simulink model "SETL2_TestLevel_2_MODEL_Training"  (R2017b)
settings: Solver=VariableStepAuto  StartTime=0.0  StopTime=25000000  MaxStep=200  RelTol=1e-3
model workspace (MAT data in the model file):
  Ba = 98.3523688074
  Br = 64.1345426034
  Bw = 39.6355439353
libraries: instrumentlib x2, svdutilitieslib x1
settings Model: Creator=Bruger  LastModifiedBy=koch

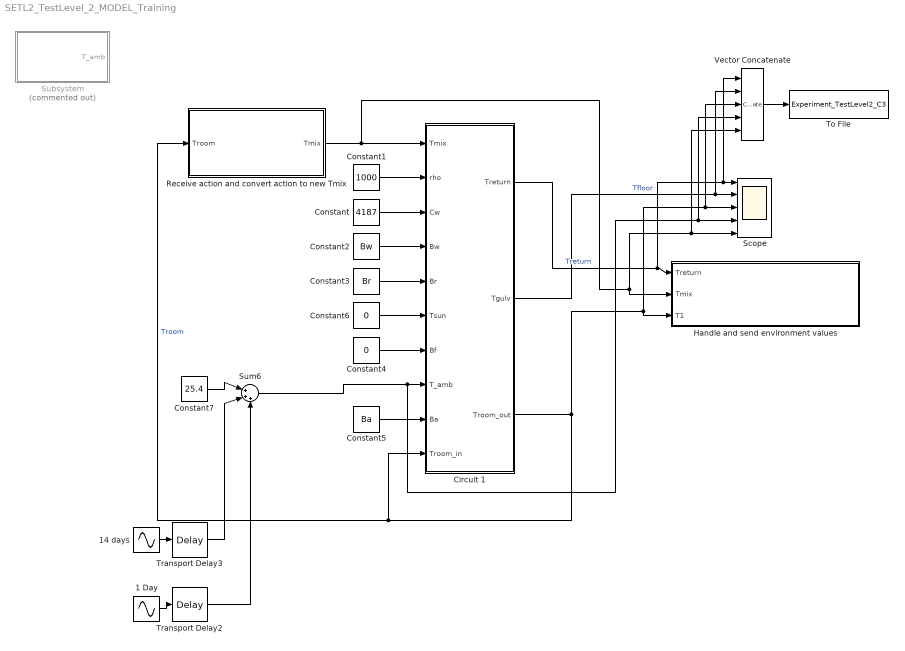
== system SETL2_TestLevel_2_MODEL_Training ==
  1 Day : Sin  Frequency=0.00014  SampleTime=0
  14 days : Sin  Frequency=0.00007272205216643  SampleTime=0
  Circuit 1 : Subsystem
  Constant : Constant  Value=4187
  Constant1 : Constant  Value=1000
  Constant2 : Constant  Value=Bw
  Constant3 : Constant  Value=Br
  Constant4 : Constant  Value=0
  Constant5 : Constant  Value=Ba
  Constant6 : Constant  Value=0
  Constant7 : Constant  Value=25.4
  Handle and send environment values : Subsystem
  Receive action and convert action to new Tmix : Subsystem
  Scope : Scope  NumInputPorts=5
  Subsystem : Subsystem  Commented=on
  Sum6 : Sum  Inputs=|+++
  To File : ToFile  Filename=Experiment_TestLevel2_C3  SaveFormat=Timeseries
  Transport Delay2 : TransportDelay  DelayTime=4000000
  Transport Delay3 : TransportDelay  DelayTime=3000000
  Vector Concatenate : Concatenate  NumInputs=5
  wires:
  Circuit 1/1(Treturn) -> Vector Concatenate/1, Scope/1, Handle and send environment values/1(Treturn)  "Treturn"
  Circuit 1/3(Troom_out) -> Vector Concatenate/3, Scope/3, Handle and send environment values/3(T1), Receive action and convert action to new Tmix/1(Troom), Circuit 1/10(Troom_in)  "Troom"
  Constant1/1 -> Circuit 1/2(rho)
  Constant/1 -> Circuit 1/3(Cw)
  Constant2/1 -> Circuit 1/4(Bw)
  Constant3/1 -> Circuit 1/5(Br)
  Constant6/1 -> Circuit 1/6(Tsun)
  Constant4/1 -> Circuit 1/7(Bf)
  Constant5/1 -> Circuit 1/9(Ba)
  Receive action and convert action to new Tmix/1(Tmix) -> Vector Concatenate/5, Scope/5, Handle and send environment values/2(Tmix), Circuit 1/1(Tmix)
  Vector Concatenate/1 -> To File/1
  Circuit 1/2(Tgulv) -> Vector Concatenate/2, Scope/2  "Tfloor"
  Transport Delay3/1 -> Sum6/2
  Constant7/1 -> Sum6/1
  14 days/1 -> Transport Delay3/1
  1 Day/1 -> Transport Delay2/1
  Transport Delay2/1 -> Sum6/3
  Sum6/1 -> Vector Concatenate/4, Scope/4, Circuit 1/8(T_amb)

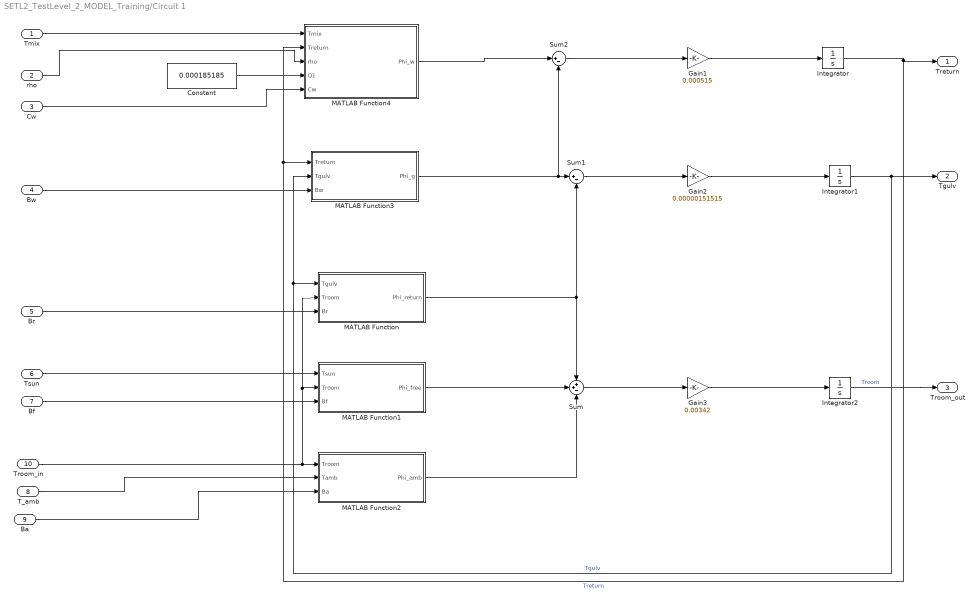
== system SETL2_TestLevel_2_MODEL_Training/Circuit 1 ==
  Tmix : Inport
  rho : Inport  Port=2
  Cw : Inport  Port=3
  Bw : Inport  Port=4
  Br : Inport  Port=5
  Tsun : Inport  Port=6
  Bf : Inport  Port=7
  T_amb : Inport  Port=8
  Ba : Inport  Port=9
  Troom_in : Inport  Port=10
  Constant : Constant  Value=0.000185185
  Gain1 : Gain  Gain=0.000515
  Gain2 : Gain  Gain=0.00000151515
  Gain3 : Gain  Gain=0.00342
  Integrator : Integrator  InitialCondition=25.5
  Integrator1 : Integrator  InitialCondition=25.5
  Integrator2 : Integrator  InitialCondition=25.5
  MATLAB Function : MATLAB Function  TreatAsAtomicUnit=on
  MATLAB Function1 : MATLAB Function  TreatAsAtomicUnit=on
  MATLAB Function2 : MATLAB Function  TreatAsAtomicUnit=on
  MATLAB Function3 : MATLAB Function  TreatAsAtomicUnit=on
  MATLAB Function4 : MATLAB Function  TreatAsAtomicUnit=on
  Sum : Sum  Inputs=++-
  Sum1 : Sum  Inputs=|+-
  Sum2 : Sum  Inputs=|+-
  Treturn : Outport
  Tgulv : Outport  Port=2
  Troom_out : Outport  Port=3
  wires:
  MATLAB Function1/1(Phi_free) -> Sum/2
  MATLAB Function4/1(Phi_w) -> Sum2/1
  Constant/1 -> MATLAB Function4/4(Q1)
  MATLAB Function2/1(Phi_amb) -> Sum/3
  Sum2/1 -> Gain1/1
  Bf/1 -> MATLAB Function1/3(Bf)
  Integrator1/1 -> MATLAB Function/1(Tgulv), MATLAB Function3/2(Tgulv), Tgulv/1  "Tgulv"
  Integrator2/1 -> Troom_out/1  "Troom"
  MATLAB Function3/1(Phi_g) -> Sum2/2, Sum1/1
  MATLAB Function/1(Phi_return) -> Sum/1, Sum1/2
  Bw/1 -> MATLAB Function3/3(Bw)
  Cw/1 -> MATLAB Function4/5(Cw)
  rho/1 -> MATLAB Function4/3(rho)
  Sum1/1 -> Gain2/1
  Gain1/1 -> Integrator/1
  Gain2/1 -> Integrator1/1
  Integrator/1 -> MATLAB Function4/2(Treturn), MATLAB Function3/1(Treturn), Treturn/1  "Treturn"
  Tsun/1 -> MATLAB Function1/1(Tsun)
  Gain3/1 -> Integrator2/1
  Ba/1 -> MATLAB Function2/3(Ba)
  Br/1 -> MATLAB Function/3(Br)
  Sum/1 -> Gain3/1
  Troom_in/1 -> MATLAB Function2/1(Troom), MATLAB Function/2(Troom), MATLAB Function1/2(Troom)
  Tmix/1 -> MATLAB Function4/1(Tmix)
  T_amb/1 -> MATLAB Function2/2(Tamb)

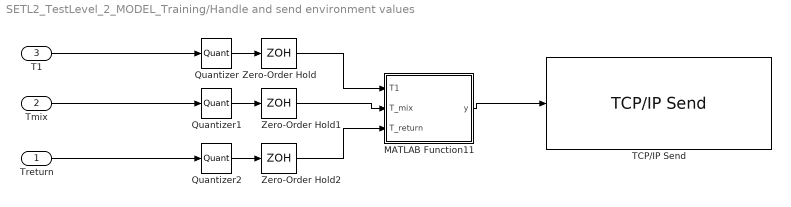
== system SETL2_TestLevel_2_MODEL_Training/Handle and send environment values ==
  Treturn : Inport
  Tmix : Inport  Port=2
  T1 : Inport  Port=3
  MATLAB Function11 : MATLAB Function  TreatAsAtomicUnit=on
  Quantizer : Quantizer  QuantizationInterval=0.01
  Quantizer1 : Quantizer  QuantizationInterval=0.01
  Quantizer2 : Quantizer  QuantizationInterval=0.01
  TCP/IP Send : instrumentlib/TCP//IP Send  Priority=2  Host=localhost  Port=50001  EnableBlockingMode=on  Timeout=10  ByteOrder=LittleEndian
      settings: SourceProductName=Instrument Control Toolbox
  Zero-Order Hold : ZeroOrderHold  SampleTime=-1
  Zero-Order Hold1 : ZeroOrderHold  SampleTime=-1
  Zero-Order Hold2 : ZeroOrderHold  SampleTime=-1
  wires:
  Quantizer1/1 -> Zero-Order Hold1/1
  Quantizer/1 -> Zero-Order Hold/1
  Quantizer2/1 -> Zero-Order Hold2/1
  Zero-Order Hold1/1 -> MATLAB Function11/2(T_mix)
  Zero-Order Hold/1 -> MATLAB Function11/1(T1)
  Zero-Order Hold2/1 -> MATLAB Function11/3(T_return)
  MATLAB Function11/1(y) -> TCP/IP Send/1
  Tmix/1 -> Quantizer1/1
  T1/1 -> Quantizer/1
  Treturn/1 -> Quantizer2/1

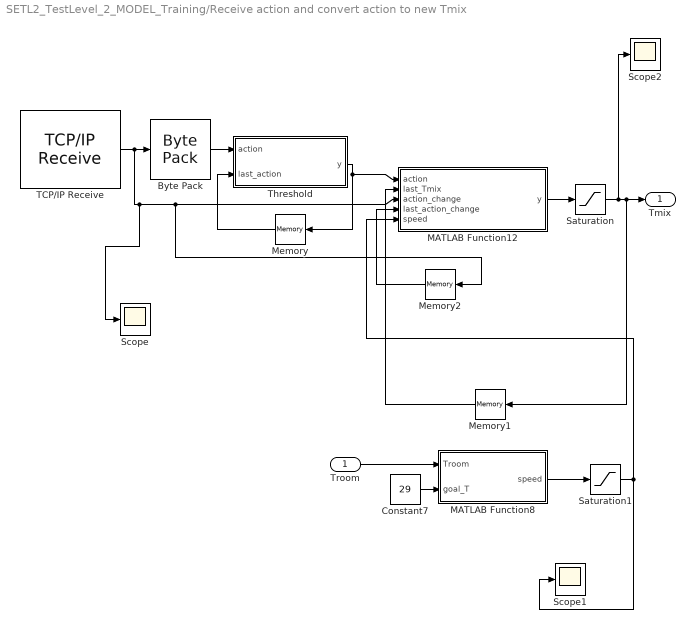
== system SETL2_TestLevel_2_MODEL_Training/Receive action and convert action to new Tmix ==
  Troom : Inport
  Byte Pack : svdutilitieslib/Byte Pack  datatypes={'uint8'}  byteAlign=1  blockPlatform=arduinoert
      settings: SourceProductName=Simulink Support Package for Arduino Hardware  SourceProductBaseCode=ARDUINO
  Constant7 : Constant  Value=29
  MATLAB Function12 : MATLAB Function  TreatAsAtomicUnit=on
  MATLAB Function8 : MATLAB Function  TreatAsAtomicUnit=on
  Memory : Memory
  Memory1 : Memory  InitialCondition=24
  Memory2 : Memory
  Saturation : Saturate  UpperLimit=60  LowerLimit=24
  Saturation1 : Saturate  UpperLimit=0.8  LowerLimit=0.005
  Scope : Scope
  Scope1 : Scope
  Scope2 : Scope
  TCP/IP Receive : instrumentlib/TCP//IP Receive  Host=localhost  Port=50000  DataSize=[1 1]  EnableBlockingMode=on  Timeout=15  SampleTime=50  DataType=uint8  ByteOrder=BigEndian
      settings: SourceProductName=Instrument Control Toolbox
  Threshold : MATLAB Function  TreatAsAtomicUnit=on
  Tmix : Outport
  wires:
  MATLAB Function12/1(y) -> Saturation/1
  TCP/IP Receive/1 -> Scope/1, Memory2/1, MATLAB Function12/3(action_change), Byte Pack/1
  Threshold/1(y) -> MATLAB Function12/1(action), Memory/1
  MATLAB Function8/1(speed) -> Saturation1/1
  Saturation1/1 -> Scope1/1, MATLAB Function12/5(speed)
  Memory/1 -> Threshold/2(last_action)
  Saturation/1 -> Scope2/1, Tmix/1, Memory1/1
  Byte Pack/1 -> Threshold/1(action)
  Constant7/1 -> MATLAB Function8/2(goal_T)
  Memory1/1 -> MATLAB Function12/2(last_Tmix)
  Troom/1 -> MATLAB Function8/1(Troom)
  Memory2/1 -> MATLAB Function12/4(last_action_change)

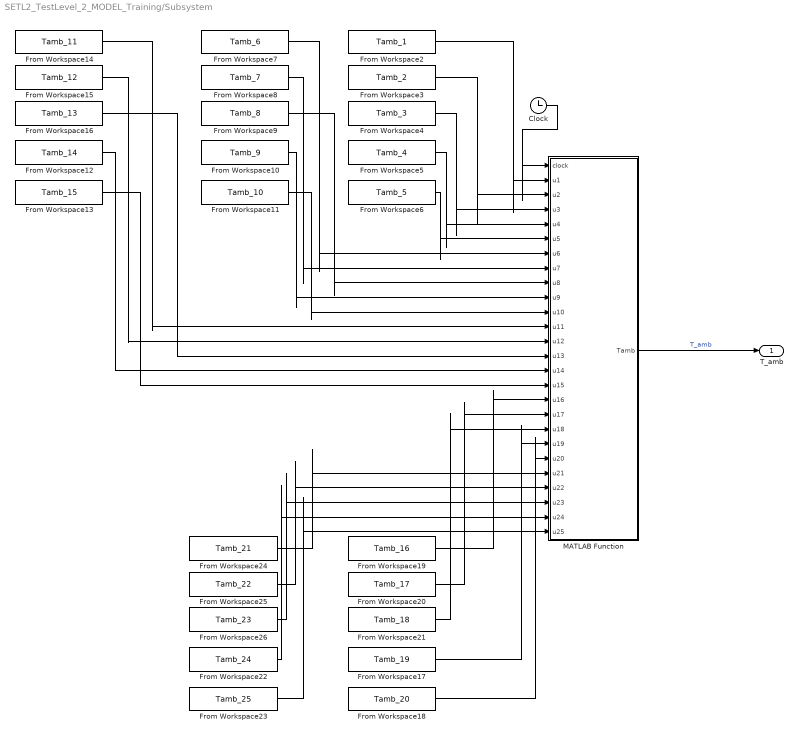
== system SETL2_TestLevel_2_MODEL_Training/Subsystem ==
  Clock : Clock
  From Workspace10 : FromWorkspace  VariableName=Tamb_9  SampleTime=0
  From Workspace11 : FromWorkspace  VariableName=Tamb_10  SampleTime=0
  From Workspace12 : FromWorkspace  VariableName=Tamb_14  SampleTime=0
  From Workspace13 : FromWorkspace  VariableName=Tamb_15  SampleTime=0
  From Workspace14 : FromWorkspace  VariableName=Tamb_11  SampleTime=0
  From Workspace15 : FromWorkspace  VariableName=Tamb_12  SampleTime=0
  From Workspace16 : FromWorkspace  VariableName=Tamb_13  SampleTime=0
  From Workspace17 : FromWorkspace  VariableName=Tamb_19  SampleTime=0
  From Workspace18 : FromWorkspace  VariableName=Tamb_20  SampleTime=0
  From Workspace19 : FromWorkspace  VariableName=Tamb_16  SampleTime=0
  From Workspace2 : FromWorkspace  VariableName=Tamb_1  SampleTime=0
  From Workspace20 : FromWorkspace  VariableName=Tamb_17  SampleTime=0
  From Workspace21 : FromWorkspace  VariableName=Tamb_18  SampleTime=0
  From Workspace22 : FromWorkspace  VariableName=Tamb_24  SampleTime=0
  From Workspace23 : FromWorkspace  VariableName=Tamb_25  SampleTime=0
  From Workspace24 : FromWorkspace  VariableName=Tamb_21  SampleTime=0
  From Workspace25 : FromWorkspace  VariableName=Tamb_22  SampleTime=0
  From Workspace26 : FromWorkspace  VariableName=Tamb_23  SampleTime=0
  From Workspace3 : FromWorkspace  VariableName=Tamb_2  SampleTime=0
  From Workspace4 : FromWorkspace  VariableName=Tamb_3  SampleTime=0
  From Workspace5 : FromWorkspace  VariableName=Tamb_4  SampleTime=0
  From Workspace6 : FromWorkspace  VariableName=Tamb_5  SampleTime=0
  From Workspace7 : FromWorkspace  VariableName=Tamb_6  SampleTime=0
  From Workspace8 : FromWorkspace  VariableName=Tamb_7  SampleTime=0
  From Workspace9 : FromWorkspace  VariableName=Tamb_8  SampleTime=0
  MATLAB Function : MATLAB Function  TreatAsAtomicUnit=on
  T_amb : Outport
  wires:
  Clock/1 -> MATLAB Function/1(clock)
  From Workspace3/1 -> MATLAB Function/3(u2)
  MATLAB Function/1(Tamb) -> T_amb/1  "T_amb"
  From Workspace22/1 -> MATLAB Function/25(u24)
  From Workspace6/1 -> MATLAB Function/6(u5)
  From Workspace4/1 -> MATLAB Function/4(u3)
  From Workspace7/1 -> MATLAB Function/7(u6)
  From Workspace18/1 -> MATLAB Function/21(u20)
  From Workspace16/1 -> MATLAB Function/14(u13)
  From Workspace15/1 -> MATLAB Function/13(u12)
  From Workspace5/1 -> MATLAB Function/5(u4)
  From Workspace9/1 -> MATLAB Function/9(u8)
  From Workspace13/1 -> MATLAB Function/16(u15)
  From Workspace11/1 -> MATLAB Function/11(u10)
  From Workspace14/1 -> MATLAB Function/12(u11)
  From Workspace20/1 -> MATLAB Function/18(u17)
  From Workspace12/1 -> MATLAB Function/15(u14)
  From Workspace10/1 -> MATLAB Function/10(u9)
  From Workspace25/1 -> MATLAB Function/23(u22)
  From Workspace24/1 -> MATLAB Function/22(u21)
  From Workspace26/1 -> MATLAB Function/24(u23)
  From Workspace8/1 -> MATLAB Function/8(u7)
  From Workspace19/1 -> MATLAB Function/17(u16)
  From Workspace23/1 -> MATLAB Function/26(u25)
  From Workspace21/1 -> MATLAB Function/19(u18)
  From Workspace17/1 -> MATLAB Function/20(u19)
  From Workspace2/1 -> MATLAB Function/2(u1)

== matlab function SETL2_TestLevel_2_MODEL_Training/Circuit 1/MATLAB Function1 ==
  data: Tsun input; Phi_free output; Troom input; Bf input
function Phi_free = fcn(Tsun,Troom,Bf)

Phi_free = Bf * ( Tsun-Troom)

== matlab function SETL2_TestLevel_2_MODEL_Training/Circuit 1/MATLAB Function ==
  data: Tgulv input; Phi_return output; Troom input; Br input
function Phi_return = fcn(Tgulv,Troom,Br)

Phi_return = Br * ( Tgulv-Troom)

== matlab function SETL2_TestLevel_2_MODEL_Training/Circuit 1/MATLAB Function2 ==
  data: Troom input; Tamb input; Phi_amb output; Ba input
function Phi_amb = fcn(Troom,Tamb,Ba)

Phi_amb = Ba * ( Troom-Tamb)

== matlab function SETL2_TestLevel_2_MODEL_Training/Circuit 1/MATLAB Function3 ==
  data: Treturn input; Tgulv input; Phi_g output; Bw input
function Phi_g= fcn(Treturn,Tgulv,Bw)

Phi_g = Bw * ( Treturn-Tgulv)

== matlab function SETL2_TestLevel_2_MODEL_Training/Circuit 1/MATLAB Function4 ==
  data: Tmix input; Treturn input; Phi_w output; rho input; Q1 input; Cw input
function Phi_w= fcn(Tmix,Treturn,rho,Q1,Cw)

Phi_w = rho*Q1 *Cw* ( Tmix-Treturn)

== matlab function SETL2_TestLevel_2_MODEL_Training/Subsystem/MATLAB Function ==
  data: clock input; Tamb output; u1 input; u2 input; u3 input; u4 input; u5 input; u6 input; u7 input; u8 input; u9 input; u10 input; u11 input; u12 input; u13 input; u14 input; u15 input; u16 input; u17 input; u18 input; u19 input; u20 input; u21 input; u22 input; u23 input; u24 input; u25 input
function Tamb = fcn(clock, u1, u2, u3, u4, u5, u6, u7, u8, u9, u10, u11, u12, u13, u14, u15, u16, u17, u18, u19, u20, u21, u22, u23, u24, u25)

if clock <= 1604445
    Tamb = 25.4375;
elseif 1604445 < clock <= 1604445*2
    Tamb = u2;
elseif 1604445*2 < clock <= 1604445*3
    Tamb = u3;
elseif 1604445*3 < clock <= 1604445*4
    Tamb = u4;
elseif 1604445*4 < clock <= 1604445*5
    Tamb = u5;
elseif 1604445*5 < clock <= 1604445*6
    Tamb = u6;
elseif 1604445*6 < clock <= 1604445*7
    Tamb = u7;
elseif 1604445*7 < clock <= 1604445*8
    Tamb = u8;
elseif 1604445*8 < clock <= 1604445*9
    Tamb = u9;
elseif 1604445*9 < clock <= 1604445*10
    Tamb = u10;
elseif 1604445*10 < clock <= 1604445*11
    Tamb = u11;
elseif 1604445*11 < clock <= 1604445*12
    Tamb = u12;
elseif 1604445*12 < clock <= 1604445*13
    Tamb = u13;
elseif 1604445*13 < clock <= 1604445*14
    Tamb = u14;
elseif 1604445*14 < clock <= 1604445*15
    Tamb = u15;
elseif 1604445*15 < clock <= 1604445*16
    Tamb = u16;
elseif 1604445*16 < clock <= 1604445*17
    Tamb = u17;
elseif 1604445*17 < clock <= 1604445*18
    Tamb = u18;
elseif 1604445*18 < clock <= 1604445*19
    Tamb = u19;
elseif 1604445*19 < clock <= 1604445*20
    Tamb = u20;
elseif 1604445*20 < clock <= 1604445*21
    Tamb = u21;
elseif 1604445*21 < clock <= 1604445*22
    Tamb = u22;
elseif 1604445*22 < clock <= 1604445*23
    Tamb = u23;
elseif 1604445*23 < clock <= 1604445*24
    Tamb = u24;
elseif 1604445*24 < clock <= 1604445*25
    Tamb = u25;





else 
    Tamb = 0;
end

== matlab function SETL2_TestLevel_2_MODEL_Training/Receive action and convert action to new Tmix/MATLAB Function8 ==
  data: speed output; Troom input; goal_T input
function speed = fcn(Troom, goal_T)

if goal_T > 0 && Troom > 0
    speed = abs(goal_T - Troom)*1.5;
else 
    speed = 0.1;
end

if speed < 0.03
    speed =0.03;
end

== matlab function SETL2_TestLevel_2_MODEL_Training/Handle and send environment values/MATLAB Function11 ==
  data: T1 input; y output; T_mix input; T_return input
function y = fcn(T1, T_mix, T_return)


y = [T1,4.5,4.6,4.7,T_mix,T_return];

== matlab function SETL2_TestLevel_2_MODEL_Training/Receive action and convert action to new Tmix/MATLAB Function12 ==
  data: action input; y output; last_Tmix input; action_change input; last_action_change input; speed input
function y = fcn(action, last_Tmix, action_change,last_action_change, speed)

%Only make change if a action is received by the TCP/IP receiver
if action_change > last_action_change 
    k = 1;
else
    k = 0;
end


if action == 30
    y = 45;
elseif action < 2 && k>0
    y = last_Tmix;
    k = 0;
elseif 1 < action && action < 3 && k>0
    y = last_Tmix - speed;
    k = 0;
elseif 2 < action && k>0
    y = last_Tmix+speed;
    k = 0;
elseif action > 20
    y = action;
else
    y = last_Tmix;
end

== matlab function SETL2_TestLevel_2_MODEL_Training/Receive action and convert action to new Tmix/Threshold ==
  data: action input; y output; last_action input
function y  = fcn(action,last_action)

action = double(action);
% zero is not a option so
if action > 0
    y = action;
else
    y = last_action;
end
